simulink model "Crane_LQR_disc_noisy"  (R2018a)
settings: Solver=VariableStepAuto  StartTime=0.0  StopTime=30  RelTol=1e-3
undefined symbols (not defined in the file): A, Ao, B, Bo, C, Co, F, L, RefFWD, sigbuilder_block, xinit
libraries: simulink x1, dspfdesign x1
settings Model: Creator=tcbooij  LastModifiedBy=nemezis
settings CodeAppCC: StateflowObjectComments=on

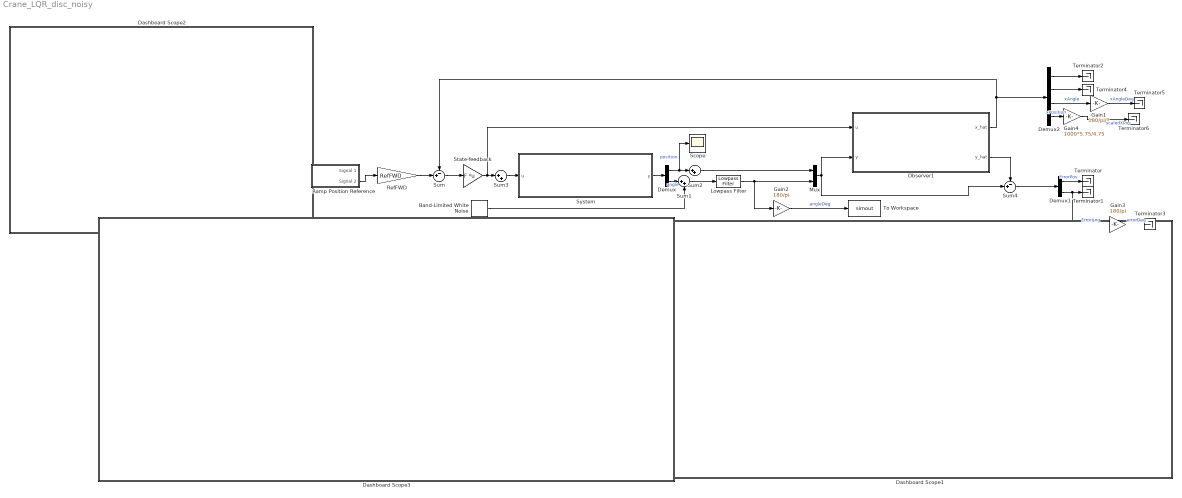
== system Crane_LQR_disc_noisy ==
  Band-Limited White Noise : simulink/Sources/Band-Limited White Noise  Cov=[0.00001]  Ts=0.01  seed=[23341]
  Dashboard Scope1 : Subsystem  DialogController=hmiCreateDDGDialog  IsWebBlock=on  mask(MWDashboardBlock){webBlockId=94ce42f8-c4e1-41da-82c1-a31c02963333, webBlockType=sdiscope, ShowInitialText=on, HMISrcModelName=Crane_LQR_disc_noisy}
      mask prompts: webBlockId "WebBlock Id"; webBlockType "WebBlock Type"; HMISrcModelName "Source Model"
      mask help: SimulinkHMI:dialogs:HMIScopeDialogDesc
      mask Help: helpview([docroot '/mapfiles/simulink.map'], 'hmi_scope')
      mask Display:
      | if strcmp(get_param(bdroot(gcb),'BlockDiagramType'), 'library')
      |     image([(matlabroot) '/toolbox/simulink/hmi/icons/DashboardScope.png']);
      | end
  Dashboard Scope2 : Subsystem  DialogController=hmiCreateDDGDialog  IsWebBlock=on  mask(MWDashboardBlock){webBlockId=2571b827-ae84-4a1c-bc36-e22ee194435d, webBlockType=sdiscope, ShowInitialText=on, HMISrcModelName=Crane_LQR_disc_noisy}
      mask prompts: webBlockId "WebBlock Id"; webBlockType "WebBlock Type"; HMISrcModelName "Source Model"
      mask help: SimulinkHMI:dialogs:HMIScopeDialogDesc
      mask Help: helpview([docroot '/mapfiles/simulink.map'], 'hmi_scope')
      mask Display:
      | if strcmp(get_param(bdroot(gcb),'BlockDiagramType'), 'library')
      |     image([(matlabroot) '/toolbox/simulink/hmi/icons/DashboardScope.png']);
      | end
  Dashboard Scope3 : Subsystem  DialogController=hmiCreateDDGDialog  IsWebBlock=on  mask(MWDashboardBlock){webBlockId=8652e169-738a-43eb-99bc-869d98056901, webBlockType=sdiscope, ShowInitialText=on, HMISrcModelName=Crane_LQR_disc_noisy}
      mask prompts: webBlockId "WebBlock Id"; webBlockType "WebBlock Type"; HMISrcModelName "Source Model"
      mask help: SimulinkHMI:dialogs:HMIScopeDialogDesc
      mask Help: helpview([docroot '/mapfiles/simulink.map'], 'hmi_scope')
      mask Display:
      | if strcmp(get_param(bdroot(gcb),'BlockDiagramType'), 'library')
      |     image([(matlabroot) '/toolbox/simulink/hmi/icons/DashboardScope.png']);
      | end
  Demux : Demux  Outputs=2
  Demux1 : Demux  Outputs=2
  Demux2 : Demux
  Gain1 : Gain  Gain=180/pi/2
  Gain2 : Gain  Gain=180/pi
  Gain3 : Gain  Gain=180/pi
  Gain4 : Gain  Gain=1000*5.75/4.75
  Lowpass Filter : dspfdesign/Lowpass Filter  FilterType=IIR  DesignForMinimumOrder=on  FilterOrder=50  PassbandFrequency=1e2  StopbandFrequency=2e2  PassbandRipple=0.1  StopbandAttenuation=80  InheritSampleRate=off  SampleRate=44100  SimulateUsing=Interpreted execution  roundingMode=Floor  coeffsDataTypeStr=fixdt(1,16)
  Mux : Mux  Inputs=2
  Observer1 : Subsystem
  Ramp Position Reference : Subsystem  Tag=STV Subsys  LoadFcn=sigbuilder_block('load',[403.5 83.25 565.5 401.25 ]);  StartFcn=sigbuilder_block('start');  StopFcn=sigbuilder_block('stop');  ClipboardFcn=sigbuilder_block('clipboard');  mask(Sigbuilder block){tuvar=[0:10]}
      mask help: Simulink:masks:SigbuilderBlock_MD
      mask init:
      | if ~strcmp(get_param(bdroot(gcbh),'SimulationStatus'),'stopped') tuvar = sigbuilder_block('maskInit'); end
      settings: CopyFcn=sigbuilder_block('copy');  DeleteFcn=sigbuilder_block('delete');  ModelCloseFcn=sigbuilder_block('modelClose');  PreSaveFcn=sigbuilder_block('preSave');  PauseFcn=sigbuilder_block('pause');  ContinueFcn=sigbuilder_block('continue');  NameChangeFcn=sigbuilder_block('namechange');  OpenFcn=sigbuilder_block('open',[403.5 83.25 565.5 401.25 ]);  CloseFcn=sigbuilder_block('close');
      mask Display: plot(0, 0, 100, 100,[2, 2, 32, 32, 2], [68, 8, 8, 68, 68],[32, 2], [38, 38], [32, 19, 2],[53, 60, 44], [32, 17, 17, 2],[16, 16, 31, 31]);txt = getActiveGroup(gcbh);text(2, 100, txt,'verticalAlignment', 'top');
  RefFWD : Gain  Gain=RefFWD
  Scope : Scope
  State-feedback : Gain  Gain=F  Multiplication=Matrix(K*u)
  Sum : Sum  Inputs=-+|
  Sum1 : Sum  Inputs=|++
  Sum2 : Sum  Inputs=|++
  Sum3 : Sum  Inputs=|++
  Sum4 : Sum  Inputs=-+|
  System : Subsystem
  Terminator{,1..6} (7 alike) : Terminator
  To Workspace : ToWorkspace  VariableName=simout  SaveFormat=Timeseries  SampleTime=-1
  wires:
  System/1(y) -> Demux/1
  Mux/1 -> Observer1/2(y), Sum4/2
  Demux1/2 -> Gain3/1, Terminator1/1  "ErrorAng"
  Demux1/1 -> Terminator/1  "ErrorPos"
  Gain2/1 -> To Workspace/1  "angleDeg"
  Gain3/1 -> Terminator3/1  "errorDeg"
  Demux/2 -> Sum1/1  "angle"
  Demux/1 -> Scope/1, Sum2/1  "position"
  Sum2/1 -> Mux/1
  Sum3/1 -> System/1(u)
  Sum4/1 -> Demux1/1
  Observer1/1(x_hat) -> Sum/1, Demux2/1
  Observer1/2(y_hat) -> Sum4/1
  Demux2/4 -> Gain4/1  "xPosition"
  Demux2/3 -> Gain1/1  "xAngle"
  Demux2/2 -> Terminator4/1
  Demux2/1 -> Terminator2/1
  Gain1/1 -> Terminator5/1  "xAngleDeg"
  Gain4/1 -> Terminator6/1  "scaledXPos"
  RefFWD/1 -> Sum/2
  Sum/1 -> State-feedback/1
  State-feedback/1 -> Observer1/1(u), Sum3/1
  Sum1/1 -> Lowpass Filter/1
  Lowpass Filter/1 -> Gain2/1, Mux/2
  Ramp Position Reference/2(Signal 2) -> RefFWD/1
  Band-Limited White Noise/1 -> Sum1/2

== system Crane_LQR_disc_noisy/Dashboard Scope1 ==

== system Crane_LQR_disc_noisy/Dashboard Scope2 ==

== system Crane_LQR_disc_noisy/Dashboard Scope3 ==

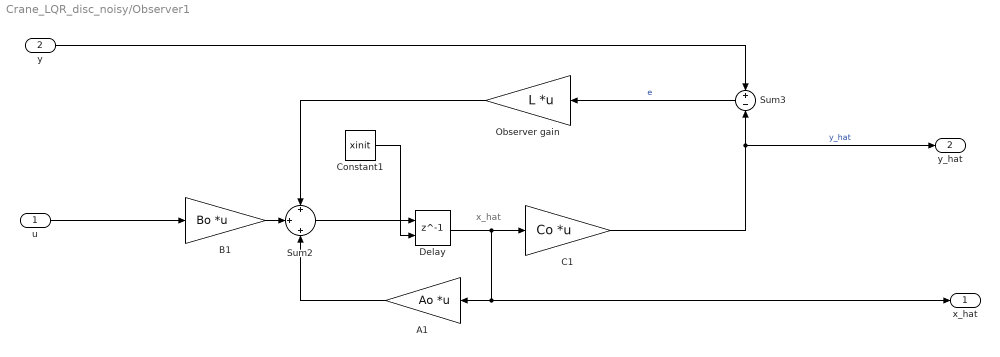
== system Crane_LQR_disc_noisy/Observer1 ==
  note: x_hat
  u : Inport
  y : Inport  Port=2
  A1 : Gain  Gain=Ao  Multiplication=Matrix(K*u)
  B1 : Gain  Gain=Bo  Multiplication=Matrix(K*u)
  C1 : Gain  Gain=Co  Multiplication=Matrix(K*u)
  Constant1 : Constant  Value=xinit
  Delay : Delay  DelayLength=1  InitialConditionSource=Input port
      settings: InputPortMap=u0,p4
  Observer gain : Gain  Gain=L  Multiplication=Matrix(K*u)
  Sum2 : Sum  Inputs=+|+|+
  Sum3 : Sum  Inputs=+|-
  x_hat : Outport
  y_hat : Outport  Port=2
  wires:
  Constant1/1 -> Delay/2
  Sum2/1 -> Delay/1
  Delay/1 -> C1/1, A1/1, x_hat/1
  Observer gain/1 -> Sum2/1
  C1/1 -> Sum3/2, y_hat/1  "y_hat"
  u/1 -> B1/1
  B1/1 -> Sum2/2
  A1/1 -> Sum2/3
  y/1 -> Sum3/1
  Sum3/1 -> Observer gain/1  "e"

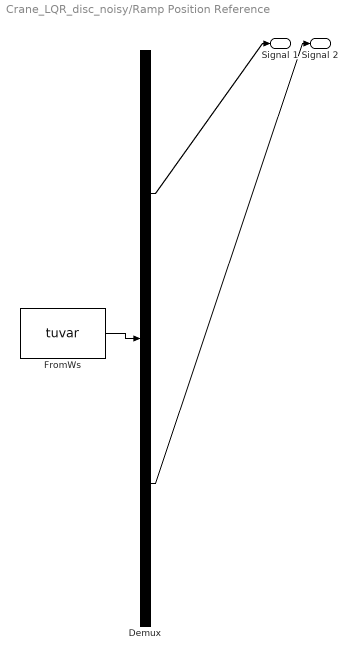
== system Crane_LQR_disc_noisy/Ramp Position Reference ==
  Demux : Demux  Tag=STV Demux  Outputs=2
  FromWs : FromWorkspace  Tag=STV FromWs  VariableName=tuvar  SampleTime=0
      SigBuilderData=|
      | common.afterFinalStr = 'Extrapolate'
      | common.sampleTime = 0
      | dataSet.timeRange = [0 30]
      | dataSet.name = 'Group 1'
      | sbobj.Groups.Name = 'Group 1'
      | sbobj.Groups.Signals(1).Name = 'Signal 1'
      | sbobj.Groups.Signals(1).XData = [0 0.222222222222 0.444444444444 0.666666666667 0.888888888889 1.11111111111 1.33333333333 1.55555555556 1.77777777778 2 2.22222222222 2.44444444444 2.66666666667 2.88888888889 3.11111111111 3.33333333333 3.55555555556 3.77777777778 4 4.22222222222 4.44444444444 4.66666666667 4.88888888889 5.11111111111 5.33333333333 5.55555555556 5.77777777778 6 6.22222222222 6.44444444444 6.66666666667 6.88888888889 7.11111111111 7.33333333333 7.55555555556 7.77777777778 8 8.22222222222 8.44444444444 8.66666666667 8.88888888889 9.11111111111 9.33333333333 9.55555555556 9.77777777778 10 10.2222222222 10.4444444444 10.6666666667 10.8888888889 11.1111111111 11.3333333333 11.5555555556 11.7777777778 12 12.2222222222 12.4444444444 12.6666666667 12.8888888889 13.1111111111 13.3333333333 13.5555555556 13.7777777778 14 14.2222222222 14.4444444444 14.6666666667 14.8888888889 15.1111111111 15.3333333333 15.5555555556 15.7777777778 16 16.2222222222 16.4444444444 16.6666666667 16.8888888889 17.1111111111 17.3333333333 17.5555555556 17.7777777778 18 18.2222222222 18.4444444444 18.6666666667 18.8888888889 19.1111111111 19.3333333333 19.5555555556 19.7777777778 20 20.2222222222 20.4444444444 20.6666666667 20.8888888889 21.1111111111 21.3333333333 21.5555555556 21.7777777778 22 22.2222222222 22.4444444444 22.6666666667 22.8888888889 23.1111111111 23.3333333333 23.5555555556 23.7777777778 24 24.2222222222 24.4444444444 24.6666666667 24.8888888889 25.1111111111 25.3333333333 25.5555555556 25.7777777778 26 26.2222222222 26.4444444444 26.6666666667 26.8888888889 27.1111111111 27.3333333333 27.5555555556 27.7777777778 28 28.2222222222 28.4444444444 28.6666666667 28.8888888889 29.1111111111 29.3333333333 29.5555555556 29.7777777778 30]
      | sbobj.Groups.Signals(1).YData = [0 1.28557521937 1.96961550602 1.73205080757 0.684040286651 -0.684040286651 -1.73205080757 -1.96961550602 -1.28557521937 0 1.28557521937 1.96961550602 1.73205080757 0.684040286651 -0.684040286651 -1.73205080757 -1.96961550602 -1.28557521937 0 1.28557521937 1.96961550602 1.73205080757 0.684040286651 -0.684040286651 -1.73205080757 -1.96961550602 -1.28557521937 0 1.28557521937 1.96961550602 1.73205080757 0.684040286651 -0.684040286651 -1.73205080757 -1.96961550602 -1.28557521937 0 1.28557521937 1.96961550602 1.73205080757 0.684040286651 -0.684040286651 -1.73205080757 -1.96961550602 -1.28557521937 0 1.28557521937 1.96961550602 1.73205080757 0.684040286651 -0.684040286651 -1.73205080757 -1.96961550602 -1.28557521937 0 1.28557521937 1.96961550602 1.73205080757 0.684040286651 -0.684040286651 -1.73205080757 -1.96961550602 -1.28557521937 0 1.28557521937 1.96961550602 1.73205080757 0.684040286651 -0.684040286651 -1.73205080757 -1.96961550602 -1.28557521937 0 1.28557521937 1.96961550602 1.73205080757 0.684040286651 -0.684040286651 -1.73205080757 -1.96961550602 -1.28557521937 0 1.28557521937 1.96961550602 1.73205080757 0.684040286651 -0.684040286651 -1.73205080757 -1.96961550602 -1.28557521937 0 1.28557521937 1.96961550602 1.73205080757 0.684040286651 -0.684040286651 -1.73205080757 -1.96961550602 -1.28557521937 0 1.28557521937 1.96961550602 1.73205080757 0.684040286651 -0.684040286651 -1.73205080757 -1.96961550602 -1.28557521937 0 1.28557521937 1.96961550602 1.73205080757 0.684040286651 -0.684040286651 -1.73205080757 -1.96961550602 -1.28557521937 0 1.28557521937 1.96961550602 1.73205080757 0.684040286651 -0.684040286651 -1.73205080757 -1.96961550602 -1.28557521937 0 1.28557521937 1.96961550602 1.73205080757 0.684040286651 -0.684040286651 -1.73205080757 -1.96961550602 -1.28557521937 0]
      | sbobj.Groups.Signals(2).Name = 'Signal 2'
      | sbobj.Groups.Signals(2).XData = [0 2.5 5 7.5 10 12.5 15 17.5 20 22.5 25 27.5 30]
      | sbobj.Groups.Signals(2).YData = [0 0 1 1 0 0 -1 -1 0 0 1 1 0]
      | sbobj.Groups.TimeRange = [0 30]
  Signal 1 : Outport  Tag=STV Outport
  Signal 2 : Outport  Tag=STV Outport  Port=2
  wires:
  FromWs/1 -> Demux/1
  Demux/1 -> Signal 1/1
  Demux/2 -> Signal 2/1

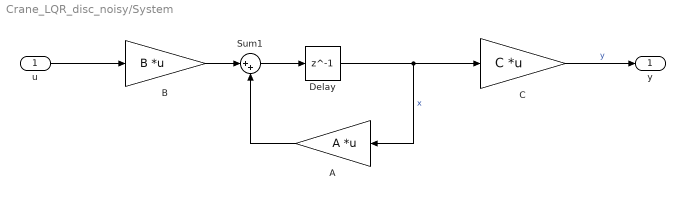
== system Crane_LQR_disc_noisy/System ==
  u : Inport
  A : Gain  Gain=A  Multiplication=Matrix(K*u)
  B : Gain  Gain=B  Multiplication=Matrix(K*u)
  C : Gain  Gain=C  Multiplication=Matrix(K*u)
  Delay : Delay  DelayLength=1
  Sum1 : Sum  Inputs=|++
  y : Outport
  wires:
  Sum1/1 -> Delay/1
  u/1 -> B/1
  C/1 -> y/1  "y"
  Delay/1 -> A/1, C/1  "x"
  A/1 -> Sum1/2
  B/1 -> Sum1/1
